simulink model "Ex_Sep_2020_B"  (R2022b)
settings: Solver=VariableStepAuto  StartTime=0.0  StopTime=150  RelTol=1e-3
settings Model: Creator=rrilo  LastModifiedBy=rrilo

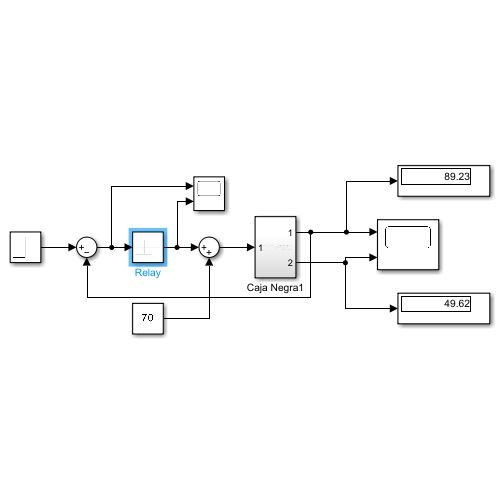
[thumbnail: Simulink's stored preview of the top-level diagram]
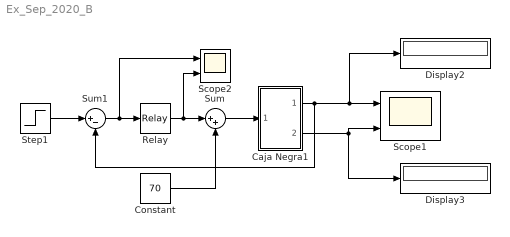
== system Ex_Sep_2020_B ==
  Caja Negra1 : Subsystem
  Constant : Constant  Value=70
  Display2 : Display
  Display3 : Display
  Relay : Relay  OnOutputValue=5  OffOutputValue=-5
  Scope1 : Scope  NumInputPorts=2
  Scope2 : Scope  NumInputPorts=2
  Step1 : Step  After=90  SampleTime=0
  Sum : Sum  Inputs=|++
  Sum1 : Sum  Inputs=|+-
  wires:
  Caja Negra1/2(Output) -> Scope1/2, Display3/1
  Constant/1 -> Sum/2
  Step1/1 -> Sum1/1
  Sum1/1 -> Scope2/1, Relay/1
  Relay/1 -> Scope2/2, Sum/1
  Caja Negra1/1(Out1) -> Scope1/1, Display2/1, Sum1/2
  Sum/1 -> Caja Negra1/1(In1)

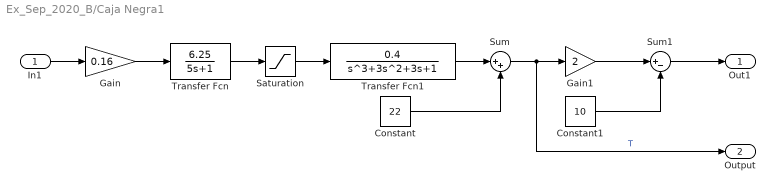
== system Ex_Sep_2020_B/Caja Negra1 ==
  In1 : Inport
  Constant : Constant  Value=22
  Constant1 : Constant  Value=10
  Gain : Gain  Gain=0.16
  Gain1 : Gain  Gain=2
  Saturation : Saturate  UpperLimit=100  LowerLimit=0
  Sum : Sum  Inputs=|++
  Sum1 : Sum  Inputs=|+-
  Transfer Fcn : TransferFcn  Numerator=[6.25]  Denominator=[5 1]
  Transfer Fcn1 : TransferFcn  Numerator=[0.4]  Denominator=[1 3 3 1]
  Out1 : Outport
  Output : Outport  Port=2
  wires:
  In1/1 -> Gain/1
  Sum1/1 -> Out1/1
  Transfer Fcn/1 -> Saturation/1
  Saturation/1 -> Transfer Fcn1/1
  Constant1/1 -> Sum1/2
  Transfer Fcn1/1 -> Sum/1
  Sum/1 -> Gain1/1, Output/1  "T"
  Gain1/1 -> Sum1/1
  Gain/1 -> Transfer Fcn/1
  Constant/1 -> Sum/2
